simulink model "Zero_Perturb_MPPT_Live"  (R2026a)
settings: Solver=ode23t  StopTime=2  FixedStep=1e-6  MaxStep=1e-5
libraries: nesl_utility x6, ee_lib x5, fl_lib x5, simulink x1
(part 2 of 2)

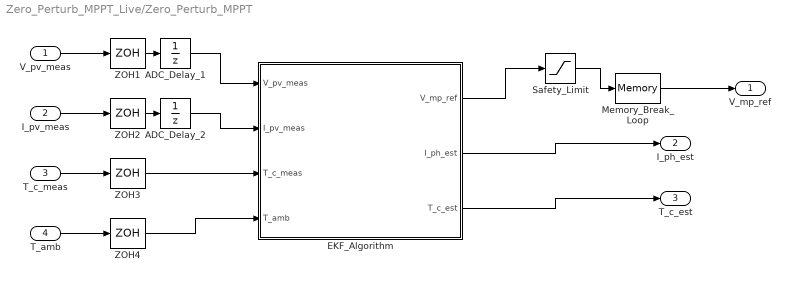
== system Zero_Perturb_MPPT_Live/Zero_Perturb_MPPT ==
  V_pv_meas : Inport
  I_pv_meas : Inport  Port=2
  T_c_meas : Inport  Port=3
  T_amb : Inport  Port=4
  ADC_Delay_1 : UnitDelay  SampleTime=-1
  ADC_Delay_2 : UnitDelay  SampleTime=-1
  EKF_Algorithm : MATLAB Function  TreatAsAtomicUnit=on
  Memory_Break_Loop : Memory  InitialCondition=17.5  InheritSampleTime=on
  Safety_Limit : Saturate  UpperLimit=21.0  LowerLimit=8.0
  ZOH{1..4} (4 alike) : ZeroOrderHold  SampleTime=0.02
  V_mp_ref : Outport
  I_ph_est : Outport  Port=2
  T_c_est : Outport  Port=3
  wires:
  V_pv_meas/1 -> ZOH1/1
  I_pv_meas/1 -> ZOH2/1
  T_c_meas/1 -> ZOH3/1
  T_amb/1 -> ZOH4/1
  ZOH3/1 -> EKF_Algorithm/3(T_c_meas)
  ZOH4/1 -> EKF_Algorithm/4(T_amb)
  EKF_Algorithm/1(V_mp_ref) -> Safety_Limit/1
  EKF_Algorithm/2(I_ph_est) -> I_ph_est/1
  EKF_Algorithm/3(T_c_est) -> T_c_est/1
  Safety_Limit/1 -> Memory_Break_Loop/1
  Memory_Break_Loop/1 -> V_mp_ref/1
  ZOH1/1 -> ADC_Delay_1/1
  ADC_Delay_1/1 -> EKF_Algorithm/1(V_pv_meas)
  ZOH2/1 -> ADC_Delay_2/1
  ADC_Delay_2/1 -> EKF_Algorithm/2(I_pv_meas)

== matlab function Zero_Perturb_MPPT_Live/Zero_Perturb_MPPT/EKF_Algorithm ==
  data: V_pv_meas input; V_mp_ref output; I_pv_meas input; T_c_meas input; T_amb input; I_ph_est output; T_c_est output
function [V_mp_ref, I_ph_est, T_c_est] = EKF_Algorithm(V_pv_meas, I_pv_meas, T_c_meas, T_amb)
    persistent x_est P_est is_initialized Param

    if isempty(is_initialized)
        Param.Voc = 21.6; Param.Vmp = 17.5; Param.I0 = 1.2e-9;
        Param.Rs = 0.35; Param.Rsh = 600.0; Param.n = 1.25; Param.Ts = 0.02;
        Param.Ns = 36; % 36 series cells in a 10W panel
        Param.Q = [1e-5, 0.0; 0.0, 1e-3];
        Param.R = [1e-3, 0.0; 0.0, 0.20];
        x_est = [0.65; 25.0];
        P_est = [1e-2, 0.0; 0.0, 1.0];
        is_initialized = true;
    end

    q = 1.60217663e-19; k = 1.380649e-23; tau_th = 300.0; Ts = Param.Ts;
    
    % State Prediction
    A = [1.0, 0.0; 0.0, 1.0 - (Ts / tau_th)];
    x_pred = [x_est(1); x_est(2) + (Ts / tau_th) * (T_amb - x_est(2))];
    P_pred = A * P_est * A' + Param.Q;
    
    % Scaled thermal voltage for 36 cells
    T_k_pred = x_pred(2) + 273.15; T0_k = 298.15; Eg = 1.12;
    I0_T = Param.I0 * ((T_k_pred / T0_k)^3) * exp((q * Eg / (Param.n * k)) * (1.0/T0_k - 1.0/T_k_pred));
    Vt_panel = Param.Ns * (k * T_k_pred) / q;
    
    % Bounded junction calculation
    V_junc = V_pv_meas + I_pv_meas * Param.Rs;
    exp_arg = min(max(V_junc / (Param.n * Vt_panel), -20.0), 25.0);
    
    h1 = x_pred(1) - I0_T * (exp(exp_arg) - 1.0) - (V_junc / Param.Rsh);
    h2 = x_pred(2);
    
    % Measurement Update
    C = [1.0, 0.0; 0.0, 1.0];
    innov = [I_pv_meas - h1; T_c_meas - h2];
    S = C * P_pred * C' + Param.R;
    K = (P_pred * C') / S;
    
    x_est = x_pred + K * innov;
    x_est(1) = max(x_est(1), 0.0); x_est(2) = max(x_est(2), -20.0);
    
    I_mat = eye(2);
    P_est = (I_mat - K * C) * P_pred * (I_mat - K * C)' + K * Param.R * K';
    
    % Lambert-W Root Extraction for Analytical MPP
    T_k_hat = x_est(2) + 273.15;
    Vt_panel_hat = Param.Ns * (k * T_k_hat) / q;
    I0_hat = Param.I0 * ((T_k_hat / T0_k)^3) * exp((q * Eg / (Param.n * k)) * (1.0/T0_k - 1.0/T_k_hat));
    
    z = exp(1.0) * (x_est(1) + I0_hat) / I0_hat;
    lz = log(z); llz = log(lz); w = lz - llz + (llz / lz);
    
    for iter = 1:4
        ew = exp(w); f = w * ew - z;
        f1 = ew * (w + 1.0); f2 = ew * (w + 2.0);
        w = w - (f / (f1 - (f * f2) / (2.0 * f1)));
    end
    
    V_mp_ref = Param.n * Vt_panel_hat * (w - 1.0) - x_est(1) * Param.Rs;
    V_mp_ref = min(max(V_mp_ref, 5.0), Param.Voc);
    I_ph_est = x_est(1);
    T_c_est = x_est(2);
end
